simulink model "lqr_test"  (R2023a)
settings: Solver=VariableStepAuto  StartTime=0.0  StopTime=10  RelTol=1e-3  EnableMultiTasking=on
undefined symbols (not defined in the file or in its folder): DiscIntNeverNeededParam
libraries: aausat3_lib x1
settings Model: Creator=jn  LastModifiedBy=jacobel-omar
settings SolverCC: AlgebraicLoopSolver=TrustRegion
settings DataIOCC: SaveFormat=Array  ReturnWorkspaceOutputs=off
settings OptimizationCC: LifeSpan=inf
settings DebuggingCC: SolverPrmCheckMsg=warning  UnconnectedInputMsg=warning  UnconnectedOutputMsg=warning  UnconnectedLineMsg=warning  AllowSymbolicDim=off  SFUnexpectedBacktrackingDiag=warning  SFNoUnconditionalDefaultTransitionDiag=warning  SFExecutionAtInitializationDiag=none  ArithmeticOperatorsInVariantConditions=warning
settings ModelReferenceCC: EnableRefExpFcnMdlSchedulingChecks=on  PropagateSignalLabelsOutOfModel=off
settings SFSimCC: SimUseLocalCustomCode=off  CustomCodeUndefinedFunction=UseInterfaceOnly
settings RTWCC: RTWUseLocalCustomCode=off
settings CodeAppCC: StateflowObjectComments=on
settings GRTTargetCC: TargetLangStandard=C89/C90 (ANSI)
settings ConfigComp: CovMetricSettings=dw  CovSaveCumulativeToWorkspaceVar=on  CovSaveSingleToWorkspaceVar=on  CovExternalEMLEnable=off  CovSFcnEnable=off

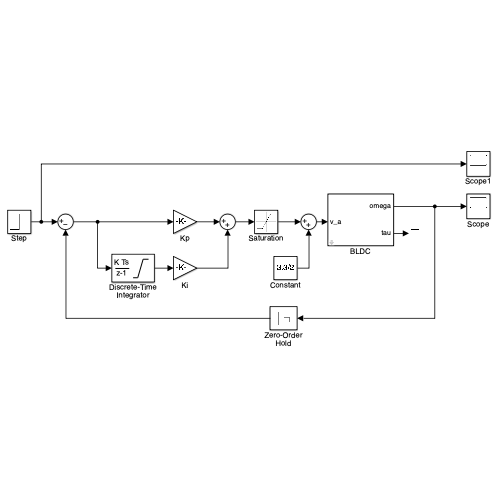
[thumbnail: Simulink's stored preview of the top-level diagram]
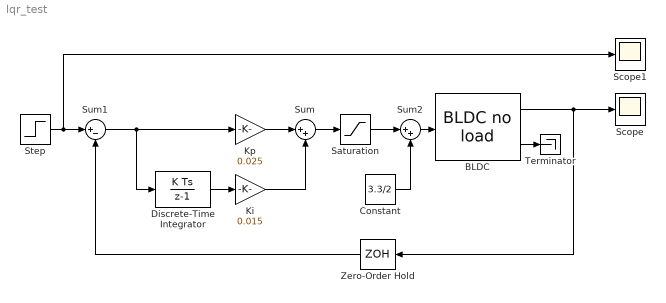
== system lqr_test ==
  BLDC : aausat3_lib/Actuator Emulation/BLDC no load  J_rotor=0.237e-7  J_rw=0.336e-6  Ra=4.44  L=0.12e-3  Kt=1.81e-3  Ke=1.81e-3  b=6.3895e-08  Vcc=3.3  init_omega=800
      settings: SourceProductName=AAUSAT3
  Constant : Constant  Value=3.3/2
  Discrete-Time Integrator : DiscreteIntegrator  SampleTime=1/20  LimitOutput=on  UpperSaturationLimit=100  LowerSaturationLimit=-100  ICPrevOutput=DiscIntNeverNeededParam  ICPrevScaledInput=DiscIntNeverNeededParam
  Ki : Gain  Gain=0.015
  Kp : Gain  Gain=0.025
  Saturation : Saturate  UpperLimit=3.3/2  LowerLimit=-3.3/2
  Scope : Scope
  Scope1 : Scope
  Step : Step  Before=800  After=1600  SampleTime=1
  Sum : Sum  Inputs=|++
  Sum1 : Sum  Inputs=|+-
  Sum2 : Sum  Inputs=|++
  Terminator : Terminator
  Zero-Order Hold : ZeroOrderHold  SampleTime=1/20
  wires:
  BLDC/1 -> Scope/1, Zero-Order Hold/1
  BLDC/2 -> Terminator/1
  Step/1 -> Scope1/1, Sum1/1
  Saturation/1 -> Sum2/1
  Zero-Order Hold/1 -> Sum1/2
  Sum1/1 -> Discrete-Time Integrator/1, Kp/1
  Discrete-Time Integrator/1 -> Ki/1
  Kp/1 -> Sum/1
  Ki/1 -> Sum/2
  Sum/1 -> Saturation/1
  Sum2/1 -> BLDC/1
  Constant/1 -> Sum2/2
